simulink model "gm_spec_avg_CRD_vs"  (R2025b)
settings: Solver=FixedStepDiscrete  StartTime=0.0  StopTime=0.0005  FixedStep=1.66666666666667e-08  RelTol=1e-3
undefined symbols (not defined in the file or in its folder): chirp_counts, chirp_outputs, clk, clk_enable, FFT_LENGTH, Fs, h, reset, specAvg
libraries: simulink x30, hdlmdlgenlib x4, dsphdlsigops2 x2, dsphdlxfrm2 x1, hdlsllib x1, vivadosimlib x1
(part 2 of 2)

== system gm_spec_avg_CRD_vs/Digital Spectrometer from Chirp DDC/Digital Spectrometer/Iteration17 ==
  xin : Inport  OutDataTypeStr=fixdt(1, 26, 15)  SampleTime=3.33333333333333e-08
  yin : Inport  Port=2  OutDataTypeStr=fixdt(1, 26, 15)  SampleTime=3.33333333333333e-08
  idx : Inport  Port=3  OutDataTypeStr=fixdt(0, 6, 0)  SampleTime=3.33333333333333e-08
  MuxX : Switch  Criteria=u2 ~= 0  Threshold="fi(0,0,1,0,\"hex\",\"0\")"  OutDataTypeStr=fixdt(1, 26, 15)  SampleTime=3.33333333333333e-08  SaturateOnIntegerOverflow=off  InputSameDT=off
  MuxY : Switch  Criteria=u2 ~= 0  Threshold="fi(0,0,1,0,\"hex\",\"0\")"  OutDataTypeStr=fixdt(1, 26, 15)  SampleTime=3.33333333333333e-08  SaturateOnIntegerOverflow=off  InputSameDT=off
  XAdder : Sum  OutDataTypeStr=fixdt(1, 26, 15)  SampleTime=3.33333333333333e-08
  XSubtractor : Sum  Inputs=+-  OutDataTypeStr=fixdt(1, 26, 15)  AccumDataTypeStr=fixdt(1, 26, 15)  SampleTime=3.33333333333333e-08
  YAdder : Sum  OutDataTypeStr=fixdt(1, 26, 15)  SampleTime=3.33333333333333e-08
  YSub : Sum  Inputs=+-  OutDataTypeStr=fixdt(1, 26, 15)  AccumDataTypeStr=fixdt(1, 26, 15)  SampleTime=3.33333333333333e-08
  compare : simulink/Logic and Bit Operations/Compare To Constant  relop=<  const=double(0)  OutDataTypeStr=boolean
  dynamic_shift : ArithShift  BitShiftNumberSource=Input port  BitShiftDirection=Right
      settings: InputPortMap=u0,p1
  dynamic_shift1 : ArithShift  BitShiftNumberSource=Input port  BitShiftDirection=Right
      settings: InputPortMap=u0,p1
  xout : Outport  OutDataTypeStr=fixdt(1, 26, 15)  SampleTime=3.33333333333333e-08
  yout : Outport  Port=2  OutDataTypeStr=fixdt(1, 26, 15)  SampleTime=3.33333333333333e-08
  wires:
  MuxX/1 -> xout/1
  MuxY/1 -> yout/1
  XAdder/1 -> MuxX/3
  XSubtractor/1 -> MuxX/1
  YSub/1 -> MuxY/3
  dynamic_shift1/1 -> XAdder/2, XSubtractor/2
  idx/1 -> dynamic_shift1/2, dynamic_shift/2
  xin/1 -> XSubtractor/1, dynamic_shift/1, XAdder/1
  compare/1 -> MuxY/2, MuxX/2
  yin/1 -> dynamic_shift1/1, compare/1, YSub/1, YAdder/1
  dynamic_shift/1 -> YSub/2, YAdder/2
  YAdder/1 -> MuxY/1

== system gm_spec_avg_CRD_vs/Digital Spectrometer from Chirp DDC/Digital Spectrometer/Iteration18 ==
  xin : Inport  OutDataTypeStr=fixdt(1, 26, 15)  SampleTime=3.33333333333333e-08
  yin : Inport  Port=2  OutDataTypeStr=fixdt(1, 26, 15)  SampleTime=3.33333333333333e-08
  idx : Inport  Port=3  OutDataTypeStr=fixdt(0, 6, 0)  SampleTime=3.33333333333333e-08
  MuxX : Switch  Criteria=u2 ~= 0  Threshold="fi(0,0,1,0,\"hex\",\"0\")"  OutDataTypeStr=fixdt(1, 26, 15)  SampleTime=3.33333333333333e-08  SaturateOnIntegerOverflow=off  InputSameDT=off
  MuxY : Switch  Criteria=u2 ~= 0  Threshold="fi(0,0,1,0,\"hex\",\"0\")"  OutDataTypeStr=fixdt(1, 26, 15)  SampleTime=3.33333333333333e-08  SaturateOnIntegerOverflow=off  InputSameDT=off
  XAdder : Sum  OutDataTypeStr=fixdt(1, 26, 15)  SampleTime=3.33333333333333e-08
  XSubtractor : Sum  Inputs=+-  OutDataTypeStr=fixdt(1, 26, 15)  AccumDataTypeStr=fixdt(1, 26, 15)  SampleTime=3.33333333333333e-08
  YAdder : Sum  OutDataTypeStr=fixdt(1, 26, 15)  SampleTime=3.33333333333333e-08
  YSub : Sum  Inputs=+-  OutDataTypeStr=fixdt(1, 26, 15)  AccumDataTypeStr=fixdt(1, 26, 15)  SampleTime=3.33333333333333e-08
  compare : simulink/Logic and Bit Operations/Compare To Constant  relop=<  const=double(0)  OutDataTypeStr=boolean
  dynamic_shift : ArithShift  BitShiftNumberSource=Input port  BitShiftDirection=Right
      settings: InputPortMap=u0,p1
  dynamic_shift1 : ArithShift  BitShiftNumberSource=Input port  BitShiftDirection=Right
      settings: InputPortMap=u0,p1
  xout : Outport  OutDataTypeStr=fixdt(1, 26, 15)  SampleTime=3.33333333333333e-08
  yout : Outport  Port=2  OutDataTypeStr=fixdt(1, 26, 15)  SampleTime=3.33333333333333e-08
  wires:
  MuxY/1 -> yout/1
  MuxX/1 -> xout/1
  YSub/1 -> MuxY/3
  YAdder/1 -> MuxY/1
  XSubtractor/1 -> MuxX/1
  XAdder/1 -> MuxX/3
  compare/1 -> MuxX/2, MuxY/2
  dynamic_shift1/1 -> XAdder/2, XSubtractor/2
  idx/1 -> dynamic_shift/2, dynamic_shift1/2
  yin/1 -> dynamic_shift1/1, compare/1, YAdder/1, YSub/1
  dynamic_shift/1 -> YAdder/2, YSub/2
  xin/1 -> XAdder/1, dynamic_shift/1, XSubtractor/1

== system gm_spec_avg_CRD_vs/Digital Spectrometer from Chirp DDC/Digital Spectrometer/Iteration19 ==
  xin : Inport  OutDataTypeStr=fixdt(1, 26, 15)  SampleTime=3.33333333333333e-08
  yin : Inport  Port=2  OutDataTypeStr=fixdt(1, 26, 15)  SampleTime=3.33333333333333e-08
  idx : Inport  Port=3  OutDataTypeStr=fixdt(0, 6, 0)  SampleTime=3.33333333333333e-08
  MuxX : Switch  Criteria=u2 ~= 0  Threshold="fi(0,0,1,0,\"hex\",\"0\")"  OutDataTypeStr=fixdt(1, 26, 15)  SampleTime=3.33333333333333e-08  SaturateOnIntegerOverflow=off  InputSameDT=off
  MuxY : Switch  Criteria=u2 ~= 0  Threshold="fi(0,0,1,0,\"hex\",\"0\")"  OutDataTypeStr=fixdt(1, 26, 15)  SampleTime=3.33333333333333e-08  SaturateOnIntegerOverflow=off  InputSameDT=off
  XAdder : Sum  OutDataTypeStr=fixdt(1, 26, 15)  SampleTime=3.33333333333333e-08
  XSubtractor : Sum  Inputs=+-  OutDataTypeStr=fixdt(1, 26, 15)  AccumDataTypeStr=fixdt(1, 26, 15)  SampleTime=3.33333333333333e-08
  YAdder : Sum  OutDataTypeStr=fixdt(1, 26, 15)  SampleTime=3.33333333333333e-08
  YSub : Sum  Inputs=+-  OutDataTypeStr=fixdt(1, 26, 15)  AccumDataTypeStr=fixdt(1, 26, 15)  SampleTime=3.33333333333333e-08
  compare : simulink/Logic and Bit Operations/Compare To Constant  relop=<  const=double(0)  OutDataTypeStr=boolean
  dynamic_shift : ArithShift  BitShiftNumberSource=Input port  BitShiftDirection=Right
      settings: InputPortMap=u0,p1
  dynamic_shift1 : ArithShift  BitShiftNumberSource=Input port  BitShiftDirection=Right
      settings: InputPortMap=u0,p1
  xout : Outport  OutDataTypeStr=fixdt(1, 26, 15)  SampleTime=3.33333333333333e-08
  yout : Outport  Port=2  OutDataTypeStr=fixdt(1, 26, 15)  SampleTime=3.33333333333333e-08
  wires:
  MuxX/1 -> xout/1
  MuxY/1 -> yout/1
  XAdder/1 -> MuxX/3
  XSubtractor/1 -> MuxX/1
  YSub/1 -> MuxY/3
  YAdder/1 -> MuxY/1
  dynamic_shift/1 -> YSub/2, YAdder/2
  xin/1 -> XSubtractor/1, dynamic_shift/1, XAdder/1
  dynamic_shift1/1 -> XAdder/2, XSubtractor/2
  idx/1 -> dynamic_shift1/2, dynamic_shift/2
  yin/1 -> YSub/1, dynamic_shift1/1, YAdder/1, compare/1
  compare/1 -> MuxY/2, MuxX/2

== system gm_spec_avg_CRD_vs/Digital Spectrometer from Chirp DDC/Digital Spectrometer/Iteration2 ==
  xin : Inport  OutDataTypeStr=fixdt(1, 26, 15)  SampleTime=3.33333333333333e-08
  yin : Inport  Port=2  OutDataTypeStr=fixdt(1, 26, 15)  SampleTime=3.33333333333333e-08
  idx : Inport  Port=3  OutDataTypeStr=fixdt(0, 6, 0)  SampleTime=3.33333333333333e-08
  MuxX : Switch  Criteria=u2 ~= 0  Threshold="fi(0,0,1,0,\"hex\",\"0\")"  OutDataTypeStr=fixdt(1, 26, 15)  SampleTime=3.33333333333333e-08  SaturateOnIntegerOverflow=off  InputSameDT=off
  MuxY : Switch  Criteria=u2 ~= 0  Threshold="fi(0,0,1,0,\"hex\",\"0\")"  OutDataTypeStr=fixdt(1, 26, 15)  SampleTime=3.33333333333333e-08  SaturateOnIntegerOverflow=off  InputSameDT=off
  XAdder : Sum  OutDataTypeStr=fixdt(1, 26, 15)  SampleTime=3.33333333333333e-08
  XSubtractor : Sum  Inputs=+-  OutDataTypeStr=fixdt(1, 26, 15)  AccumDataTypeStr=fixdt(1, 26, 15)  SampleTime=3.33333333333333e-08
  YAdder : Sum  OutDataTypeStr=fixdt(1, 26, 15)  SampleTime=3.33333333333333e-08
  YSub : Sum  Inputs=+-  OutDataTypeStr=fixdt(1, 26, 15)  AccumDataTypeStr=fixdt(1, 26, 15)  SampleTime=3.33333333333333e-08
  compare : simulink/Logic and Bit Operations/Compare To Constant  relop=<  const=double(0)  OutDataTypeStr=boolean
  dynamic_shift : ArithShift  BitShiftNumberSource=Input port  BitShiftDirection=Right
      settings: InputPortMap=u0,p1
  dynamic_shift1 : ArithShift  BitShiftNumberSource=Input port  BitShiftDirection=Right
      settings: InputPortMap=u0,p1
  xout : Outport  OutDataTypeStr=fixdt(1, 26, 15)  SampleTime=3.33333333333333e-08
  yout : Outport  Port=2  OutDataTypeStr=fixdt(1, 26, 15)  SampleTime=3.33333333333333e-08
  wires:
  MuxY/1 -> yout/1
  MuxX/1 -> xout/1
  YSub/1 -> MuxY/3
  YAdder/1 -> MuxY/1
  XAdder/1 -> MuxX/3
  compare/1 -> MuxX/2, MuxY/2
  XSubtractor/1 -> MuxX/1
  dynamic_shift1/1 -> XSubtractor/2, XAdder/2
  idx/1 -> dynamic_shift/2, dynamic_shift1/2
  dynamic_shift/1 -> YAdder/2, YSub/2
  yin/1 -> dynamic_shift1/1, YSub/1, compare/1, YAdder/1
  xin/1 -> dynamic_shift/1, XSubtractor/1, XAdder/1

== system gm_spec_avg_CRD_vs/Digital Spectrometer from Chirp DDC/Digital Spectrometer/Iteration20 ==
  xin : Inport  OutDataTypeStr=fixdt(1, 26, 15)  SampleTime=3.33333333333333e-08
  yin : Inport  Port=2  OutDataTypeStr=fixdt(1, 26, 15)  SampleTime=3.33333333333333e-08
  idx : Inport  Port=3  OutDataTypeStr=fixdt(0, 6, 0)  SampleTime=3.33333333333333e-08
  MuxX : Switch  Criteria=u2 ~= 0  Threshold="fi(0,0,1,0,\"hex\",\"0\")"  OutDataTypeStr=fixdt(1, 26, 15)  SampleTime=3.33333333333333e-08  SaturateOnIntegerOverflow=off  InputSameDT=off
  MuxY : Switch  Criteria=u2 ~= 0  Threshold="fi(0,0,1,0,\"hex\",\"0\")"  OutDataTypeStr=fixdt(1, 26, 15)  SampleTime=3.33333333333333e-08  SaturateOnIntegerOverflow=off  InputSameDT=off
  XAdder : Sum  OutDataTypeStr=fixdt(1, 26, 15)  SampleTime=3.33333333333333e-08
  XSubtractor : Sum  Inputs=+-  OutDataTypeStr=fixdt(1, 26, 15)  AccumDataTypeStr=fixdt(1, 26, 15)  SampleTime=3.33333333333333e-08
  YAdder : Sum  OutDataTypeStr=fixdt(1, 26, 15)  SampleTime=3.33333333333333e-08
  YSub : Sum  Inputs=+-  OutDataTypeStr=fixdt(1, 26, 15)  AccumDataTypeStr=fixdt(1, 26, 15)  SampleTime=3.33333333333333e-08
  compare : simulink/Logic and Bit Operations/Compare To Constant  relop=<  const=double(0)  OutDataTypeStr=boolean
  dynamic_shift : ArithShift  BitShiftNumberSource=Input port  BitShiftDirection=Right
      settings: InputPortMap=u0,p1
  dynamic_shift1 : ArithShift  BitShiftNumberSource=Input port  BitShiftDirection=Right
      settings: InputPortMap=u0,p1
  xout : Outport  OutDataTypeStr=fixdt(1, 26, 15)  SampleTime=3.33333333333333e-08
  yout : Outport  Port=2  OutDataTypeStr=fixdt(1, 26, 15)  SampleTime=3.33333333333333e-08
  wires:
  MuxY/1 -> yout/1
  MuxX/1 -> xout/1
  YSub/1 -> MuxY/3
  YAdder/1 -> MuxY/1
  XSubtractor/1 -> MuxX/1
  dynamic_shift/1 -> YAdder/2, YSub/2
  compare/1 -> MuxX/2, MuxY/2
  idx/1 -> dynamic_shift/2, dynamic_shift1/2
  yin/1 -> dynamic_shift1/1, compare/1, YAdder/1, YSub/1
  XAdder/1 -> MuxX/3
  xin/1 -> dynamic_shift/1, XSubtractor/1, XAdder/1
  dynamic_shift1/1 -> XSubtractor/2, XAdder/2

== system gm_spec_avg_CRD_vs/Digital Spectrometer from Chirp DDC/Digital Spectrometer/Iteration21 ==
  xin : Inport  OutDataTypeStr=fixdt(1, 26, 15)  SampleTime=3.33333333333333e-08
  yin : Inport  Port=2  OutDataTypeStr=fixdt(1, 26, 15)  SampleTime=3.33333333333333e-08
  idx : Inport  Port=3  OutDataTypeStr=fixdt(0, 6, 0)  SampleTime=3.33333333333333e-08
  MuxX : Switch  Criteria=u2 ~= 0  Threshold="fi(0,0,1,0,\"hex\",\"0\")"  OutDataTypeStr=fixdt(1, 26, 15)  SampleTime=3.33333333333333e-08  SaturateOnIntegerOverflow=off  InputSameDT=off
  MuxY : Switch  Criteria=u2 ~= 0  Threshold="fi(0,0,1,0,\"hex\",\"0\")"  OutDataTypeStr=fixdt(1, 26, 15)  SampleTime=3.33333333333333e-08  SaturateOnIntegerOverflow=off  InputSameDT=off
  XAdder : Sum  OutDataTypeStr=fixdt(1, 26, 15)  SampleTime=3.33333333333333e-08
  XSubtractor : Sum  Inputs=+-  OutDataTypeStr=fixdt(1, 26, 15)  AccumDataTypeStr=fixdt(1, 26, 15)  SampleTime=3.33333333333333e-08
  YAdder : Sum  OutDataTypeStr=fixdt(1, 26, 15)  SampleTime=3.33333333333333e-08
  YSub : Sum  Inputs=+-  OutDataTypeStr=fixdt(1, 26, 15)  AccumDataTypeStr=fixdt(1, 26, 15)  SampleTime=3.33333333333333e-08
  compare : simulink/Logic and Bit Operations/Compare To Constant  relop=<  const=double(0)  OutDataTypeStr=boolean
  dynamic_shift : ArithShift  BitShiftNumberSource=Input port  BitShiftDirection=Right
      settings: InputPortMap=u0,p1
  dynamic_shift1 : ArithShift  BitShiftNumberSource=Input port  BitShiftDirection=Right
      settings: InputPortMap=u0,p1
  xout : Outport  OutDataTypeStr=fixdt(1, 26, 15)  SampleTime=3.33333333333333e-08
  yout : Outport  Port=2  OutDataTypeStr=fixdt(1, 26, 15)  SampleTime=3.33333333333333e-08
  wires:
  MuxX/1 -> xout/1
  MuxY/1 -> yout/1
  XSubtractor/1 -> MuxX/1
  YSub/1 -> MuxY/3
  compare/1 -> MuxY/2, MuxX/2
  dynamic_shift1/1 -> XAdder/2, XSubtractor/2
  idx/1 -> dynamic_shift1/2, dynamic_shift/2
  XAdder/1 -> MuxX/3
  dynamic_shift/1 -> YAdder/2, YSub/2
  xin/1 -> dynamic_shift/1, XAdder/1, XSubtractor/1
  yin/1 -> dynamic_shift1/1, YSub/1, YAdder/1, compare/1
  YAdder/1 -> MuxY/1

== system gm_spec_avg_CRD_vs/Digital Spectrometer from Chirp DDC/Digital Spectrometer/Iteration22 ==
  xin : Inport  OutDataTypeStr=fixdt(1, 26, 15)  SampleTime=3.33333333333333e-08
  yin : Inport  Port=2  OutDataTypeStr=fixdt(1, 26, 15)  SampleTime=3.33333333333333e-08
  idx : Inport  Port=3  OutDataTypeStr=fixdt(0, 6, 0)  SampleTime=3.33333333333333e-08
  MuxX : Switch  Criteria=u2 ~= 0  Threshold="fi(0,0,1,0,\"hex\",\"0\")"  OutDataTypeStr=fixdt(1, 26, 15)  SampleTime=3.33333333333333e-08  SaturateOnIntegerOverflow=off  InputSameDT=off
  MuxY : Switch  Criteria=u2 ~= 0  Threshold="fi(0,0,1,0,\"hex\",\"0\")"  OutDataTypeStr=fixdt(1, 26, 15)  SampleTime=3.33333333333333e-08  SaturateOnIntegerOverflow=off  InputSameDT=off
  XAdder : Sum  OutDataTypeStr=fixdt(1, 26, 15)  SampleTime=3.33333333333333e-08
  XSubtractor : Sum  Inputs=+-  OutDataTypeStr=fixdt(1, 26, 15)  AccumDataTypeStr=fixdt(1, 26, 15)  SampleTime=3.33333333333333e-08
  YAdder : Sum  OutDataTypeStr=fixdt(1, 26, 15)  SampleTime=3.33333333333333e-08
  YSub : Sum  Inputs=+-  OutDataTypeStr=fixdt(1, 26, 15)  AccumDataTypeStr=fixdt(1, 26, 15)  SampleTime=3.33333333333333e-08
  compare : simulink/Logic and Bit Operations/Compare To Constant  relop=<  const=double(0)  OutDataTypeStr=boolean
  dynamic_shift : ArithShift  BitShiftNumberSource=Input port  BitShiftDirection=Right
      settings: InputPortMap=u0,p1
  dynamic_shift1 : ArithShift  BitShiftNumberSource=Input port  BitShiftDirection=Right
      settings: InputPortMap=u0,p1
  xout : Outport  OutDataTypeStr=fixdt(1, 26, 15)  SampleTime=3.33333333333333e-08
  yout : Outport  Port=2  OutDataTypeStr=fixdt(1, 26, 15)  SampleTime=3.33333333333333e-08
  wires:
  MuxY/1 -> yout/1
  MuxX/1 -> xout/1
  YSub/1 -> MuxY/3
  YAdder/1 -> MuxY/1
  XAdder/1 -> MuxX/3
  XSubtractor/1 -> MuxX/1
  dynamic_shift1/1 -> XSubtractor/2, XAdder/2
  idx/1 -> dynamic_shift/2, dynamic_shift1/2
  compare/1 -> MuxX/2, MuxY/2
  yin/1 -> dynamic_shift1/1, YAdder/1, compare/1, YSub/1
  dynamic_shift/1 -> YAdder/2, YSub/2
  xin/1 -> dynamic_shift/1, XSubtractor/1, XAdder/1

== system gm_spec_avg_CRD_vs/Digital Spectrometer from Chirp DDC/Digital Spectrometer/Iteration23 ==
  xin : Inport  OutDataTypeStr=fixdt(1, 26, 15)  SampleTime=3.33333333333333e-08
  yin : Inport  Port=2  OutDataTypeStr=fixdt(1, 26, 15)  SampleTime=3.33333333333333e-08
  idx : Inport  Port=3  OutDataTypeStr=fixdt(0, 6, 0)  SampleTime=3.33333333333333e-08
  MuxX : Switch  Criteria=u2 ~= 0  Threshold="fi(0,0,1,0,\"hex\",\"0\")"  OutDataTypeStr=fixdt(1, 26, 15)  SampleTime=3.33333333333333e-08  SaturateOnIntegerOverflow=off  InputSameDT=off
  MuxY : Switch  Criteria=u2 ~= 0  Threshold="fi(0,0,1,0,\"hex\",\"0\")"  OutDataTypeStr=fixdt(1, 26, 15)  SampleTime=3.33333333333333e-08  SaturateOnIntegerOverflow=off  InputSameDT=off
  XAdder : Sum  OutDataTypeStr=fixdt(1, 26, 15)  SampleTime=3.33333333333333e-08
  XSubtractor : Sum  Inputs=+-  OutDataTypeStr=fixdt(1, 26, 15)  AccumDataTypeStr=fixdt(1, 26, 15)  SampleTime=3.33333333333333e-08
  YAdder : Sum  OutDataTypeStr=fixdt(1, 26, 15)  SampleTime=3.33333333333333e-08
  YSub : Sum  Inputs=+-  OutDataTypeStr=fixdt(1, 26, 15)  AccumDataTypeStr=fixdt(1, 26, 15)  SampleTime=3.33333333333333e-08
  compare : simulink/Logic and Bit Operations/Compare To Constant  relop=<  const=double(0)  OutDataTypeStr=boolean
  dynamic_shift : ArithShift  BitShiftNumberSource=Input port  BitShiftDirection=Right
      settings: InputPortMap=u0,p1
  dynamic_shift1 : ArithShift  BitShiftNumberSource=Input port  BitShiftDirection=Right
      settings: InputPortMap=u0,p1
  xout : Outport  OutDataTypeStr=fixdt(1, 26, 15)  SampleTime=3.33333333333333e-08
  yout : Outport  Port=2  OutDataTypeStr=fixdt(1, 26, 15)  SampleTime=3.33333333333333e-08
  wires:
  MuxY/1 -> yout/1
  XAdder/1 -> MuxX/3
  MuxX/1 -> xout/1
  XSubtractor/1 -> MuxX/1
  YAdder/1 -> MuxY/1
  dynamic_shift1/1 -> XAdder/2, XSubtractor/2
  dynamic_shift/1 -> YSub/2, YAdder/2
  xin/1 -> XAdder/1, dynamic_shift/1, XSubtractor/1
  YSub/1 -> MuxY/3
  idx/1 -> dynamic_shift1/2, dynamic_shift/2
  yin/1 -> dynamic_shift1/1, YSub/1, YAdder/1, compare/1
  compare/1 -> MuxY/2, MuxX/2

== system gm_spec_avg_CRD_vs/Digital Spectrometer from Chirp DDC/Digital Spectrometer/Iteration3 ==
  xin : Inport  OutDataTypeStr=fixdt(1, 26, 15)  SampleTime=3.33333333333333e-08
  yin : Inport  Port=2  OutDataTypeStr=fixdt(1, 26, 15)  SampleTime=3.33333333333333e-08
  idx : Inport  Port=3  OutDataTypeStr=fixdt(0, 6, 0)  SampleTime=3.33333333333333e-08
  MuxX : Switch  Criteria=u2 ~= 0  Threshold="fi(0,0,1,0,\"hex\",\"0\")"  OutDataTypeStr=fixdt(1, 26, 15)  SampleTime=3.33333333333333e-08  SaturateOnIntegerOverflow=off  InputSameDT=off
  MuxY : Switch  Criteria=u2 ~= 0  Threshold="fi(0,0,1,0,\"hex\",\"0\")"  OutDataTypeStr=fixdt(1, 26, 15)  SampleTime=3.33333333333333e-08  SaturateOnIntegerOverflow=off  InputSameDT=off
  XAdder : Sum  OutDataTypeStr=fixdt(1, 26, 15)  SampleTime=3.33333333333333e-08
  XSubtractor : Sum  Inputs=+-  OutDataTypeStr=fixdt(1, 26, 15)  AccumDataTypeStr=fixdt(1, 26, 15)  SampleTime=3.33333333333333e-08
  YAdder : Sum  OutDataTypeStr=fixdt(1, 26, 15)  SampleTime=3.33333333333333e-08
  YSub : Sum  Inputs=+-  OutDataTypeStr=fixdt(1, 26, 15)  AccumDataTypeStr=fixdt(1, 26, 15)  SampleTime=3.33333333333333e-08
  compare : simulink/Logic and Bit Operations/Compare To Constant  relop=<  const=double(0)  OutDataTypeStr=boolean
  dynamic_shift : ArithShift  BitShiftNumberSource=Input port  BitShiftDirection=Right
      settings: InputPortMap=u0,p1
  dynamic_shift1 : ArithShift  BitShiftNumberSource=Input port  BitShiftDirection=Right
      settings: InputPortMap=u0,p1
  xout : Outport  OutDataTypeStr=fixdt(1, 26, 15)  SampleTime=3.33333333333333e-08
  yout : Outport  Port=2  OutDataTypeStr=fixdt(1, 26, 15)  SampleTime=3.33333333333333e-08
  wires:
  MuxX/1 -> xout/1
  MuxY/1 -> yout/1
  XSubtractor/1 -> MuxX/1
  dynamic_shift1/1 -> XAdder/2, XSubtractor/2
  YAdder/1 -> MuxY/1
  idx/1 -> dynamic_shift1/2, dynamic_shift/2
  compare/1 -> MuxY/2, MuxX/2
  xin/1 -> dynamic_shift/1, XAdder/1, XSubtractor/1
  YSub/1 -> MuxY/3
  yin/1 -> dynamic_shift1/1, compare/1, YSub/1, YAdder/1
  XAdder/1 -> MuxX/3
  dynamic_shift/1 -> YSub/2, YAdder/2

== system gm_spec_avg_CRD_vs/Digital Spectrometer from Chirp DDC/Digital Spectrometer/Iteration4 ==
  xin : Inport  OutDataTypeStr=fixdt(1, 26, 15)  SampleTime=3.33333333333333e-08
  yin : Inport  Port=2  OutDataTypeStr=fixdt(1, 26, 15)  SampleTime=3.33333333333333e-08
  idx : Inport  Port=3  OutDataTypeStr=fixdt(0, 6, 0)  SampleTime=3.33333333333333e-08
  MuxX : Switch  Criteria=u2 ~= 0  Threshold="fi(0,0,1,0,\"hex\",\"0\")"  OutDataTypeStr=fixdt(1, 26, 15)  SampleTime=3.33333333333333e-08  SaturateOnIntegerOverflow=off  InputSameDT=off
  MuxY : Switch  Criteria=u2 ~= 0  Threshold="fi(0,0,1,0,\"hex\",\"0\")"  OutDataTypeStr=fixdt(1, 26, 15)  SampleTime=3.33333333333333e-08  SaturateOnIntegerOverflow=off  InputSameDT=off
  XAdder : Sum  OutDataTypeStr=fixdt(1, 26, 15)  SampleTime=3.33333333333333e-08
  XSubtractor : Sum  Inputs=+-  OutDataTypeStr=fixdt(1, 26, 15)  AccumDataTypeStr=fixdt(1, 26, 15)  SampleTime=3.33333333333333e-08
  YAdder : Sum  OutDataTypeStr=fixdt(1, 26, 15)  SampleTime=3.33333333333333e-08
  YSub : Sum  Inputs=+-  OutDataTypeStr=fixdt(1, 26, 15)  AccumDataTypeStr=fixdt(1, 26, 15)  SampleTime=3.33333333333333e-08
  compare : simulink/Logic and Bit Operations/Compare To Constant  relop=<  const=double(0)  OutDataTypeStr=boolean
  dynamic_shift : ArithShift  BitShiftNumberSource=Input port  BitShiftDirection=Right
      settings: InputPortMap=u0,p1
  dynamic_shift1 : ArithShift  BitShiftNumberSource=Input port  BitShiftDirection=Right
      settings: InputPortMap=u0,p1
  xout : Outport  OutDataTypeStr=fixdt(1, 26, 15)  SampleTime=3.33333333333333e-08
  yout : Outport  Port=2  OutDataTypeStr=fixdt(1, 26, 15)  SampleTime=3.33333333333333e-08
  wires:
  MuxY/1 -> yout/1
  MuxX/1 -> xout/1
  YSub/1 -> MuxY/3
  XSubtractor/1 -> MuxX/1
  XAdder/1 -> MuxX/3
  compare/1 -> MuxX/2, MuxY/2
  dynamic_shift1/1 -> XSubtractor/2, XAdder/2
  idx/1 -> dynamic_shift/2, dynamic_shift1/2
  yin/1 -> YSub/1, dynamic_shift1/1, compare/1, YAdder/1
  dynamic_shift/1 -> YAdder/2, YSub/2
  xin/1 -> dynamic_shift/1, XSubtractor/1, XAdder/1
  YAdder/1 -> MuxY/1

== system gm_spec_avg_CRD_vs/Digital Spectrometer from Chirp DDC/Digital Spectrometer/Iteration5 ==
  xin : Inport  OutDataTypeStr=fixdt(1, 26, 15)  SampleTime=3.33333333333333e-08
  yin : Inport  Port=2  OutDataTypeStr=fixdt(1, 26, 15)  SampleTime=3.33333333333333e-08
  idx : Inport  Port=3  OutDataTypeStr=fixdt(0, 6, 0)  SampleTime=3.33333333333333e-08
  MuxX : Switch  Criteria=u2 ~= 0  Threshold="fi(0,0,1,0,\"hex\",\"0\")"  OutDataTypeStr=fixdt(1, 26, 15)  SampleTime=3.33333333333333e-08  SaturateOnIntegerOverflow=off  InputSameDT=off
  MuxY : Switch  Criteria=u2 ~= 0  Threshold="fi(0,0,1,0,\"hex\",\"0\")"  OutDataTypeStr=fixdt(1, 26, 15)  SampleTime=3.33333333333333e-08  SaturateOnIntegerOverflow=off  InputSameDT=off
  XAdder : Sum  OutDataTypeStr=fixdt(1, 26, 15)  SampleTime=3.33333333333333e-08
  XSubtractor : Sum  Inputs=+-  OutDataTypeStr=fixdt(1, 26, 15)  AccumDataTypeStr=fixdt(1, 26, 15)  SampleTime=3.33333333333333e-08
  YAdder : Sum  OutDataTypeStr=fixdt(1, 26, 15)  SampleTime=3.33333333333333e-08
  YSub : Sum  Inputs=+-  OutDataTypeStr=fixdt(1, 26, 15)  AccumDataTypeStr=fixdt(1, 26, 15)  SampleTime=3.33333333333333e-08
  compare : simulink/Logic and Bit Operations/Compare To Constant  relop=<  const=double(0)  OutDataTypeStr=boolean
  dynamic_shift : ArithShift  BitShiftNumberSource=Input port  BitShiftDirection=Right
      settings: InputPortMap=u0,p1
  dynamic_shift1 : ArithShift  BitShiftNumberSource=Input port  BitShiftDirection=Right
      settings: InputPortMap=u0,p1
  xout : Outport  OutDataTypeStr=fixdt(1, 26, 15)  SampleTime=3.33333333333333e-08
  yout : Outport  Port=2  OutDataTypeStr=fixdt(1, 26, 15)  SampleTime=3.33333333333333e-08
  wires:
  MuxY/1 -> yout/1
  XAdder/1 -> MuxX/3
  XSubtractor/1 -> MuxX/1
  YSub/1 -> MuxY/3
  YAdder/1 -> MuxY/1
  idx/1 -> dynamic_shift1/2, dynamic_shift/2
  MuxX/1 -> xout/1
  compare/1 -> MuxY/2, MuxX/2
  xin/1 -> dynamic_shift/1, XAdder/1, XSubtractor/1
  dynamic_shift1/1 -> XAdder/2, XSubtractor/2
  yin/1 -> dynamic_shift1/1, compare/1, YSub/1, YAdder/1
  dynamic_shift/1 -> YSub/2, YAdder/2

== system gm_spec_avg_CRD_vs/Digital Spectrometer from Chirp DDC/Digital Spectrometer/Iteration6 ==
  xin : Inport  OutDataTypeStr=fixdt(1, 26, 15)  SampleTime=3.33333333333333e-08
  yin : Inport  Port=2  OutDataTypeStr=fixdt(1, 26, 15)  SampleTime=3.33333333333333e-08
  idx : Inport  Port=3  OutDataTypeStr=fixdt(0, 6, 0)  SampleTime=3.33333333333333e-08
  MuxX : Switch  Criteria=u2 ~= 0  Threshold="fi(0,0,1,0,\"hex\",\"0\")"  OutDataTypeStr=fixdt(1, 26, 15)  SampleTime=3.33333333333333e-08  SaturateOnIntegerOverflow=off  InputSameDT=off
  MuxY : Switch  Criteria=u2 ~= 0  Threshold="fi(0,0,1,0,\"hex\",\"0\")"  OutDataTypeStr=fixdt(1, 26, 15)  SampleTime=3.33333333333333e-08  SaturateOnIntegerOverflow=off  InputSameDT=off
  XAdder : Sum  OutDataTypeStr=fixdt(1, 26, 15)  SampleTime=3.33333333333333e-08
  XSubtractor : Sum  Inputs=+-  OutDataTypeStr=fixdt(1, 26, 15)  AccumDataTypeStr=fixdt(1, 26, 15)  SampleTime=3.33333333333333e-08
  YAdder : Sum  OutDataTypeStr=fixdt(1, 26, 15)  SampleTime=3.33333333333333e-08
  YSub : Sum  Inputs=+-  OutDataTypeStr=fixdt(1, 26, 15)  AccumDataTypeStr=fixdt(1, 26, 15)  SampleTime=3.33333333333333e-08
  compare : simulink/Logic and Bit Operations/Compare To Constant  relop=<  const=double(0)  OutDataTypeStr=boolean
  dynamic_shift : ArithShift  BitShiftNumberSource=Input port  BitShiftDirection=Right
      settings: InputPortMap=u0,p1
  dynamic_shift1 : ArithShift  BitShiftNumberSource=Input port  BitShiftDirection=Right
      settings: InputPortMap=u0,p1
  xout : Outport  OutDataTypeStr=fixdt(1, 26, 15)  SampleTime=3.33333333333333e-08
  yout : Outport  Port=2  OutDataTypeStr=fixdt(1, 26, 15)  SampleTime=3.33333333333333e-08
  wires:
  MuxY/1 -> yout/1
  YSub/1 -> MuxY/3
  YAdder/1 -> MuxY/1
  XAdder/1 -> MuxX/3
  XSubtractor/1 -> MuxX/1
  compare/1 -> MuxX/2, MuxY/2
  MuxX/1 -> xout/1
  dynamic_shift1/1 -> XSubtractor/2, XAdder/2
  idx/1 -> dynamic_shift/2, dynamic_shift1/2
  yin/1 -> YSub/1, dynamic_shift1/1, compare/1, YAdder/1
  dynamic_shift/1 -> YAdder/2, YSub/2
  xin/1 -> dynamic_shift/1, XSubtractor/1, XAdder/1

== system gm_spec_avg_CRD_vs/Digital Spectrometer from Chirp DDC/Digital Spectrometer/Iteration7 ==
  xin : Inport  OutDataTypeStr=fixdt(1, 26, 15)  SampleTime=3.33333333333333e-08
  yin : Inport  Port=2  OutDataTypeStr=fixdt(1, 26, 15)  SampleTime=3.33333333333333e-08
  idx : Inport  Port=3  OutDataTypeStr=fixdt(0, 6, 0)  SampleTime=3.33333333333333e-08
  MuxX : Switch  Criteria=u2 ~= 0  Threshold="fi(0,0,1,0,\"hex\",\"0\")"  OutDataTypeStr=fixdt(1, 26, 15)  SampleTime=3.33333333333333e-08  SaturateOnIntegerOverflow=off  InputSameDT=off
  MuxY : Switch  Criteria=u2 ~= 0  Threshold="fi(0,0,1,0,\"hex\",\"0\")"  OutDataTypeStr=fixdt(1, 26, 15)  SampleTime=3.33333333333333e-08  SaturateOnIntegerOverflow=off  InputSameDT=off
  XAdder : Sum  OutDataTypeStr=fixdt(1, 26, 15)  SampleTime=3.33333333333333e-08
  XSubtractor : Sum  Inputs=+-  OutDataTypeStr=fixdt(1, 26, 15)  AccumDataTypeStr=fixdt(1, 26, 15)  SampleTime=3.33333333333333e-08
  YAdder : Sum  OutDataTypeStr=fixdt(1, 26, 15)  SampleTime=3.33333333333333e-08
  YSub : Sum  Inputs=+-  OutDataTypeStr=fixdt(1, 26, 15)  AccumDataTypeStr=fixdt(1, 26, 15)  SampleTime=3.33333333333333e-08
  compare : simulink/Logic and Bit Operations/Compare To Constant  relop=<  const=double(0)  OutDataTypeStr=boolean
  dynamic_shift : ArithShift  BitShiftNumberSource=Input port  BitShiftDirection=Right
      settings: InputPortMap=u0,p1
  dynamic_shift1 : ArithShift  BitShiftNumberSource=Input port  BitShiftDirection=Right
      settings: InputPortMap=u0,p1
  xout : Outport  OutDataTypeStr=fixdt(1, 26, 15)  SampleTime=3.33333333333333e-08
  yout : Outport  Port=2  OutDataTypeStr=fixdt(1, 26, 15)  SampleTime=3.33333333333333e-08
  wires:
  MuxX/1 -> xout/1
  MuxY/1 -> yout/1
  XAdder/1 -> MuxX/3
  XSubtractor/1 -> MuxX/1
  YAdder/1 -> MuxY/1
  dynamic_shift1/1 -> XAdder/2, XSubtractor/2
  dynamic_shift/1 -> YSub/2, YAdder/2
  idx/1 -> dynamic_shift1/2, dynamic_shift/2
  xin/1 -> dynamic_shift/1, XAdder/1, XSubtractor/1
  YSub/1 -> MuxY/3
  yin/1 -> YAdder/1, dynamic_shift1/1, YSub/1, compare/1
  compare/1 -> MuxX/2, MuxY/2

== system gm_spec_avg_CRD_vs/Digital Spectrometer from Chirp DDC/Digital Spectrometer/Iteration8 ==
  xin : Inport  OutDataTypeStr=fixdt(1, 26, 15)  SampleTime=3.33333333333333e-08
  yin : Inport  Port=2  OutDataTypeStr=fixdt(1, 26, 15)  SampleTime=3.33333333333333e-08
  idx : Inport  Port=3  OutDataTypeStr=fixdt(0, 6, 0)  SampleTime=3.33333333333333e-08
  MuxX : Switch  Criteria=u2 ~= 0  Threshold="fi(0,0,1,0,\"hex\",\"0\")"  OutDataTypeStr=fixdt(1, 26, 15)  SampleTime=3.33333333333333e-08  SaturateOnIntegerOverflow=off  InputSameDT=off
  MuxY : Switch  Criteria=u2 ~= 0  Threshold="fi(0,0,1,0,\"hex\",\"0\")"  OutDataTypeStr=fixdt(1, 26, 15)  SampleTime=3.33333333333333e-08  SaturateOnIntegerOverflow=off  InputSameDT=off
  XAdder : Sum  OutDataTypeStr=fixdt(1, 26, 15)  SampleTime=3.33333333333333e-08
  XSubtractor : Sum  Inputs=+-  OutDataTypeStr=fixdt(1, 26, 15)  AccumDataTypeStr=fixdt(1, 26, 15)  SampleTime=3.33333333333333e-08
  YAdder : Sum  OutDataTypeStr=fixdt(1, 26, 15)  SampleTime=3.33333333333333e-08
  YSub : Sum  Inputs=+-  OutDataTypeStr=fixdt(1, 26, 15)  AccumDataTypeStr=fixdt(1, 26, 15)  SampleTime=3.33333333333333e-08
  compare : simulink/Logic and Bit Operations/Compare To Constant  relop=<  const=double(0)  OutDataTypeStr=boolean
  dynamic_shift : ArithShift  BitShiftNumberSource=Input port  BitShiftDirection=Right
      settings: InputPortMap=u0,p1
  dynamic_shift1 : ArithShift  BitShiftNumberSource=Input port  BitShiftDirection=Right
      settings: InputPortMap=u0,p1
  xout : Outport  OutDataTypeStr=fixdt(1, 26, 15)  SampleTime=3.33333333333333e-08
  yout : Outport  Port=2  OutDataTypeStr=fixdt(1, 26, 15)  SampleTime=3.33333333333333e-08
  wires:
  MuxY/1 -> yout/1
  MuxX/1 -> xout/1
  YAdder/1 -> MuxY/1
  dynamic_shift/1 -> YSub/2, YAdder/2
  XAdder/1 -> MuxX/3
  idx/1 -> dynamic_shift/2, dynamic_shift1/2
  compare/1 -> MuxX/2, MuxY/2
  yin/1 -> dynamic_shift1/1, compare/1, YAdder/1, YSub/1
  XSubtractor/1 -> MuxX/1
  xin/1 -> dynamic_shift/1, XSubtractor/1, XAdder/1
  dynamic_shift1/1 -> XSubtractor/2, XAdder/2
  YSub/1 -> MuxY/3

== system gm_spec_avg_CRD_vs/Digital Spectrometer from Chirp DDC/Digital Spectrometer/Iteration9 ==
  xin : Inport  OutDataTypeStr=fixdt(1, 26, 15)  SampleTime=3.33333333333333e-08
  yin : Inport  Port=2  OutDataTypeStr=fixdt(1, 26, 15)  SampleTime=3.33333333333333e-08
  idx : Inport  Port=3  OutDataTypeStr=fixdt(0, 6, 0)  SampleTime=3.33333333333333e-08
  MuxX : Switch  Criteria=u2 ~= 0  Threshold="fi(0,0,1,0,\"hex\",\"0\")"  OutDataTypeStr=fixdt(1, 26, 15)  SampleTime=3.33333333333333e-08  SaturateOnIntegerOverflow=off  InputSameDT=off
  MuxY : Switch  Criteria=u2 ~= 0  Threshold="fi(0,0,1,0,\"hex\",\"0\")"  OutDataTypeStr=fixdt(1, 26, 15)  SampleTime=3.33333333333333e-08  SaturateOnIntegerOverflow=off  InputSameDT=off
  XAdder : Sum  OutDataTypeStr=fixdt(1, 26, 15)  SampleTime=3.33333333333333e-08
  XSubtractor : Sum  Inputs=+-  OutDataTypeStr=fixdt(1, 26, 15)  AccumDataTypeStr=fixdt(1, 26, 15)  SampleTime=3.33333333333333e-08
  YAdder : Sum  OutDataTypeStr=fixdt(1, 26, 15)  SampleTime=3.33333333333333e-08
  YSub : Sum  Inputs=+-  OutDataTypeStr=fixdt(1, 26, 15)  AccumDataTypeStr=fixdt(1, 26, 15)  SampleTime=3.33333333333333e-08
  compare : simulink/Logic and Bit Operations/Compare To Constant  relop=<  const=double(0)  OutDataTypeStr=boolean
  dynamic_shift : ArithShift  BitShiftNumberSource=Input port  BitShiftDirection=Right
      settings: InputPortMap=u0,p1
  dynamic_shift1 : ArithShift  BitShiftNumberSource=Input port  BitShiftDirection=Right
      settings: InputPortMap=u0,p1
  xout : Outport  OutDataTypeStr=fixdt(1, 26, 15)  SampleTime=3.33333333333333e-08
  yout : Outport  Port=2  OutDataTypeStr=fixdt(1, 26, 15)  SampleTime=3.33333333333333e-08
  wires:
  MuxX/1 -> xout/1
  MuxY/1 -> yout/1
  XAdder/1 -> MuxX/3
  XSubtractor/1 -> MuxX/1
  compare/1 -> MuxY/2, MuxX/2
  YAdder/1 -> MuxY/1
  dynamic_shift1/1 -> XAdder/2, XSubtractor/2
  dynamic_shift/1 -> YSub/2, YAdder/2
  idx/1 -> dynamic_shift1/2, dynamic_shift/2
  xin/1 -> dynamic_shift/1, XAdder/1, XSubtractor/1
  YSub/1 -> MuxY/3
  yin/1 -> dynamic_shift1/1, YSub/1, compare/1, YAdder/1

== system gm_spec_avg_CRD_vs/Digital Spectrometer from Chirp DDC/Digital Spectrometer/QuadrantMapper ==
  xin : Inport  OutDataTypeStr=fixdt(1, 26, 15)  SampleTime=3.33333333333333e-08
  yin : Inport  Port=2  OutDataTypeStr=fixdt(1, 26, 15)  SampleTime=3.33333333333333e-08
  DelayxAbs : UnitDelay  InitialCondition=double(0)  SampleTime=3.33333333333333e-08
  DelayyAbs : UnitDelay  InitialCondition=double(0)  SampleTime=3.33333333333333e-08
  abs : Abs  SampleTime=3.33333333333333e-08  OutDataTypeStr=fixdt(1, 26, 15)  SaturateOnIntegerOverflow=off
  abs1 : Abs  SampleTime=3.33333333333333e-08  OutDataTypeStr=fixdt(1, 26, 15)  SaturateOnIntegerOverflow=off
  dtc : hdlmdlgenlib/Buffer
  dtc1 : hdlmdlgenlib/Buffer
  mux : MultiPortSwitch  DataPortOrder=Zero-based contiguous  Inputs=2  DiagnosticForDefault=None  zeroidx=on  OutDataTypeStr=fixdt(1, 26, 15)  SampleTime=3.33333333333333e-08  SaturateOnIntegerOverflow=off  InputSameDT=off
  mux1 : MultiPortSwitch  DataPortOrder=Zero-based contiguous  Inputs=2  DiagnosticForDefault=None  zeroidx=on  OutDataTypeStr=fixdt(1, 26, 15)  SampleTime=3.33333333333333e-08  SaturateOnIntegerOverflow=off  InputSameDT=off
  relop : RelationalOperator  Operator=>  OutDataTypeStr=fixdt(0, 1, 0)  SampleTime=3.33333333333333e-08
  xout : Outport  OutDataTypeStr=fixdt(1, 26, 15)  SampleTime=3.33333333333333e-08
  yout : Outport  Port=2  OutDataTypeStr=fixdt(1, 26, 15)  SampleTime=3.33333333333333e-08
  wires:
  dtc/1 -> yout/1
  mux1/1 -> dtc1/1
  DelayyAbs/1 -> mux1/2, relop/2, mux/3
  dtc1/1 -> xout/1
  relop/1 -> mux1/1, mux/1
  DelayxAbs/1 -> mux1/3, relop/1, mux/2
  abs/1 -> DelayyAbs/1
  yin/1 -> abs/1
  abs1/1 -> DelayxAbs/1
  xin/1 -> abs1/1
  mux/1 -> dtc/1

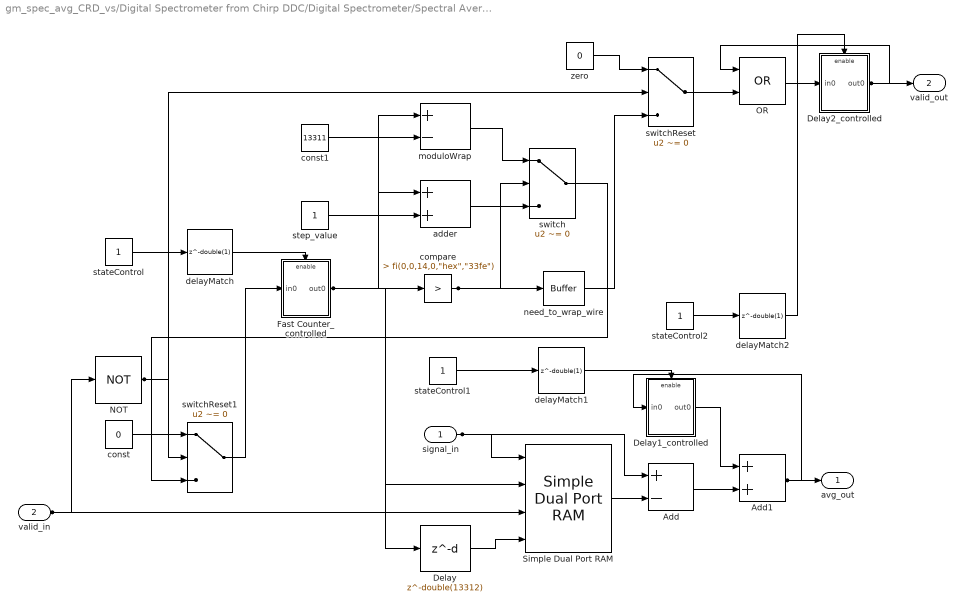
== system gm_spec_avg_CRD_vs/Digital Spectrometer from Chirp DDC/Digital Spectrometer/Spectral Averager ==
  signal_in : Inport  OutDataTypeStr=fixdt(1, 26, 15)  PortDimensions=1  SampleTime=3.33333333333333e-08
  valid_in : Inport  Port=2  OutDataTypeStr=boolean  PortDimensions=1  SampleTime=3.33333333333333e-08
  Add : Sum  Inputs=+-  OutDataTypeStr=fixdt(1, 16, 7)  AccumDataTypeStr=fixdt(1, 27, 15)  SampleTime=3.33333333333333e-08
  Add1 : Sum  OutDataTypeStr=fixdt(1, 32, 4)  AccumDataTypeStr=fixdt(1, 32, 4)  SampleTime=3.33333333333333e-08
  Delay : Delay  DelayLength=double(13312)  InitialCondition=0  SampleTime=3.33333333333333e-08
  Delay1_controlled : Subsystem
  Delay2_controlled : Subsystem
  Fast Counter_controlled : Subsystem
  NOT : Logic  Operator=NOT  Inputs=1  AllPortsSameDT=off  OutDataTypeStr=boolean  SampleTime=3.33333333333333e-08
  OR : Logic  Operator=OR  AllPortsSameDT=off  OutDataTypeStr=boolean  SampleTime=3.33333333333333e-08
  Simple Dual Port RAM : hdlsllib/HDL RAMs/Simple Dual Port RAM  ram_size=ceil(log2(specAvg))+log2(FFT_LENGTH)
  adder : Sum  OutDataTypeStr=fixdt(0, 14, 0)  AccumDataTypeStr=fixdt(0, 14, 0)  SampleTime=3.33333333333333e-08
  compare : simulink/Logic and Bit Operations/Compare To Constant  relop=>  const="fi(0,0,14,0,\"hex\",\"33fe\")"  OutDataTypeStr=boolean
  const : Constant  Value=0  VectorParams1D=off  OutDataTypeStr=fixdt(0, 14, 0)  SampleTime=3.33333333333333e-08
  const1 : Constant  Value=13311  VectorParams1D=off  OutDataTypeStr=fixdt(0, 14, 0)  SampleTime=3.33333333333333e-08
  delayMatch : Delay  DelayLength=double(1)  InitialCondition=0  SampleTime=3.33333333333333e-08
  delayMatch1 : Delay  DelayLength=double(1)  InitialCondition=0  SampleTime=3.33333333333333e-08
  delayMatch2 : Delay  DelayLength=double(1)  InitialCondition=0  SampleTime=3.33333333333333e-08
  moduloWrap : Sum  Inputs=+-  OutDataTypeStr=fixdt(0, 14, 0)  AccumDataTypeStr=fixdt(0, 14, 0)  SampleTime=3.33333333333333e-08
  need_to_wrap_wire : hdlmdlgenlib/Buffer
  stateControl : Constant  OutDataTypeStr=boolean  SampleTime=3.33333333333333e-08
  stateControl1 : Constant  OutDataTypeStr=boolean  SampleTime=3.33333333333333e-08
  stateControl2 : Constant  OutDataTypeStr=boolean  SampleTime=3.33333333333333e-08
  step_value : Constant  VectorParams1D=off  OutDataTypeStr=fixdt(0, 14, 0)  SampleTime=3.33333333333333e-08
  switch : Switch  Criteria=u2 ~= 0  Threshold="fi(0,0,1,0,\"hex\",\"0\")"  OutDataTypeStr=fixdt(0, 14, 0)  SampleTime=3.33333333333333e-08  SaturateOnIntegerOverflow=off  InputSameDT=off
  switchReset : Switch  Criteria=u2 ~= 0  Threshold="fi(0,0,1,0,\"hex\",\"0\")"  OutDataTypeStr=boolean  SampleTime=3.33333333333333e-08  SaturateOnIntegerOverflow=off  InputSameDT=off
  switchReset1 : Switch  Criteria=u2 ~= 0  Threshold="fi(0,0,1,0,\"hex\",\"0\")"  OutDataTypeStr=fixdt(0, 14, 0)  SampleTime=3.33333333333333e-08  SaturateOnIntegerOverflow=off  InputSameDT=off
  zero : Constant  Value=0  VectorParams1D=off  OutDataTypeStr=boolean  SampleTime=3.33333333333333e-08
  avg_out : Outport  SampleTime=3.33333333333333e-08
  valid_out : Outport  Port=2  SampleTime=3.33333333333333e-08  VectorParamsAs1DForOutWhenUnconnected=off
  wires:
  delayMatch2/1 -> Delay2_controlled/Enable
  OR/1 -> Delay2_controlled/1(in0)
  Add/1 -> Add1/2
  stateControl2/1 -> delayMatch2/1
  switchReset/1 -> OR/2
  Simple Dual Port RAM/1 -> Add/2
  delayMatch1/1 -> Delay1_controlled/Enable
  switch/1 -> switchReset1/3
  zero/1 -> switchReset/1
  Delay1_controlled/1(out0) -> Add1/1
  Delay/1 -> Simple Dual Port RAM/4
  stateControl1/1 -> delayMatch1/1
  compare/1 -> need_to_wrap_wire/1, switch/2
  adder/1 -> switch/3
  Delay2_controlled/1(out0) -> valid_out/1, OR/1
  moduloWrap/1 -> switch/1
  Fast Counter_controlled/1(out0) -> Delay/1, adder/1, moduloWrap/1, compare/1, Simple Dual Port RAM/2
  signal_in/1 -> Simple Dual Port RAM/1, Add/1
  need_to_wrap_wire/1 -> switchReset/3
  step_value/1 -> adder/2
  const1/1 -> moduloWrap/2
  switchReset1/1 -> Fast Counter_controlled/1(in0)
  delayMatch/1 -> Fast Counter_controlled/Enable
  const/1 -> switchReset1/1
  stateControl/1 -> delayMatch/1
  Add1/1 -> avg_out/1, Delay1_controlled/1(in0)
  NOT/1 -> switchReset1/2, switchReset/2
  valid_in/1 -> NOT/1, Simple Dual Port RAM/3

== system gm_spec_avg_CRD_vs/Digital Spectrometer from Chirp DDC/DDC/Chirp/1-D Lookup Table1 ==
  In1 : Inport
  1-D Lookup Table1 : Lookup_n-D  NumberOfTableDimensions=1  LookupTableObject=''  BreakpointsForDimension1=chirp_counts  BreakpointsForDimension1FirstPoint=10  BreakpointsForDimension2FirstPoint=10  BreakpointsForDimension1Spacing=12  BreakpointsForDimension2Spacing=12  BreakpointsForDimension1DataTypeStr=uint16  IndexSearchMethod=Evenly spaced points  Table=chirp_outputs  TableDataTypeStr=uint32  InterpMethod=Flat  InternalRulePriority=Speed  OutDataTypeStr=uint32  RndMeth=Simplest  LockScale=on
  1-D Lookup Table1_pd1 : Delay  DelayLength=1
  Out1 : Outport
  wires:
  1-D Lookup Table1_pd1/1 -> Out1/1
  1-D Lookup Table1/1 -> 1-D Lookup Table1_pd1/1
  In1/1 -> 1-D Lookup Table1/1

== system gm_spec_avg_CRD_vs/Digital Spectrometer from Chirp DDC/DDC/Chirp/Counter Limited ==
  Force to be scalar : SignalSpecification  OutDataTypeStr=uint16  Dimensions=1
  Increment Real World : Subsystem  mask(Real World Value Increment){}
      mask help: Simulink:masks:RealWorldValueIncrement_MD
      mask Display: disp('V++')
  Output : Delay  DelayLength=double(1)  InitialCondition=0  SampleTime=1.66666666666667e-08
  Wrap To Zero : Subsystem  mask(Wrap To Zero){Threshold=double(30000)}
      mask prompts: Threshold "Simulink:masks:Threshold_MP"
      mask help: Simulink:masks:WrapToZero_MD
  y : Outport  SampleTime=1.66666666666667e-08
  wires:
  Force to be scalar/1 -> Increment Real World/1(u)
  Output/1 -> Force to be scalar/1, y/1
  Increment Real World/1(y) -> Wrap To Zero/1(U)
  Wrap To Zero/1(Y) -> Output/1

== system gm_spec_avg_CRD_vs/Digital Spectrometer from Chirp DDC/Digital Spectrometer/Spectral Averager/Delay1_controlled ==
  in0 : Inport  OutDataTypeStr=fixdt(1, 32, 4)  SampleTime=3.33333333333333e-08
  stateControl : EnablePort  OutDataTypeStr=boolean
  Delay1 : Delay  DelayLength=double(512)  InitialCondition=0  SampleTime=3.33333333333333e-08
  out0 : Outport  OutDataTypeStr=fixdt(1, 32, 4)  SampleTime=3.33333333333333e-08
  wires:
  Delay1/1 -> out0/1
  in0/1 -> Delay1/1

== system gm_spec_avg_CRD_vs/Digital Spectrometer from Chirp DDC/Digital Spectrometer/Spectral Averager/Delay2_controlled ==
  in0 : Inport  OutDataTypeStr=boolean  SampleTime=3.33333333333333e-08
  stateControl : EnablePort  OutDataTypeStr=boolean
  Delay2 : Delay  DelayLength=double(1)  InitialCondition=0  SampleTime=3.33333333333333e-08
  out0 : Outport  OutDataTypeStr=boolean  SampleTime=3.33333333333333e-08
  wires:
  Delay2/1 -> out0/1
  in0/1 -> Delay2/1

== system gm_spec_avg_CRD_vs/Digital Spectrometer from Chirp DDC/Digital Spectrometer/Spectral Averager/Fast Counter_controlled ==
  in0 : Inport  OutDataTypeStr=fixdt(0, 14, 0)  SampleTime=3.33333333333333e-08
  stateControl : EnablePort  OutDataTypeStr=boolean
  Fast Counter : Delay  DelayLength=double(1)  InitialCondition=0  SampleTime=3.33333333333333e-08
  out0 : Outport  OutDataTypeStr=fixdt(0, 14, 0)  SampleTime=3.33333333333333e-08
  wires:
  Fast Counter/1 -> out0/1
  in0/1 -> Fast Counter/1

== system gm_spec_avg_CRD_vs/Digital Spectrometer from Chirp DDC/DDC/Chirp/Counter Limited/Increment Real World ==
  u : Inport  OutDataTypeStr=uint16  SampleTime=1.66666666666667e-08
  FixPt Constant : Constant  DisableCoverage=on  OutDataTypeStr=uint16  SampleTime=-1
  FixPt Sum1 : Sum  OutDataTypeStr=uint16  InputSameDT=on  LockScale=on
  y : Outport  SampleTime=1.66666666666667e-08
  wires:
  FixPt Constant/1 -> FixPt Sum1/2
  u/1 -> FixPt Sum1/1
  FixPt Sum1/1 -> y/1

== system gm_spec_avg_CRD_vs/Digital Spectrometer from Chirp DDC/DDC/Chirp/Counter Limited/Wrap To Zero ==
  note: U(k)
  U : Inport  OutDataTypeStr=uint16  SampleTime=1.66666666666667e-08
  Constant : Constant  DisableCoverage=on  Value=0  OutDataTypeStr=uint16  SampleTime=-1
  FixPt Switch : Switch  Criteria=u2 > Threshold  Threshold=Threshold  OutDataTypeStr=uint16  ZeroCross=off  SaturateOnIntegerOverflow=off  InputSameDT=off
  Y : Outport  SampleTime=1.66666666666667e-08  InitialOutput=0
  wires:
  FixPt Switch/1 -> Y/1
  U/1 -> FixPt Switch/2, FixPt Switch/3
  Constant/1 -> FixPt Switch/1
